simulink model "singlephaseasynchronousmotorwithFC"  (Simulink 7.3)
settings: Solver=ode45  StartTime=0.0  StopTime=0.5  RelTol=1e-3
undefined symbols (not defined in the file): Capacitor, Start
libraries: powerlib x8, simulink x2, electricdrivelib x1
settings Model: Creator=BRIG7Q  LastModifiedBy=BRIG7Q

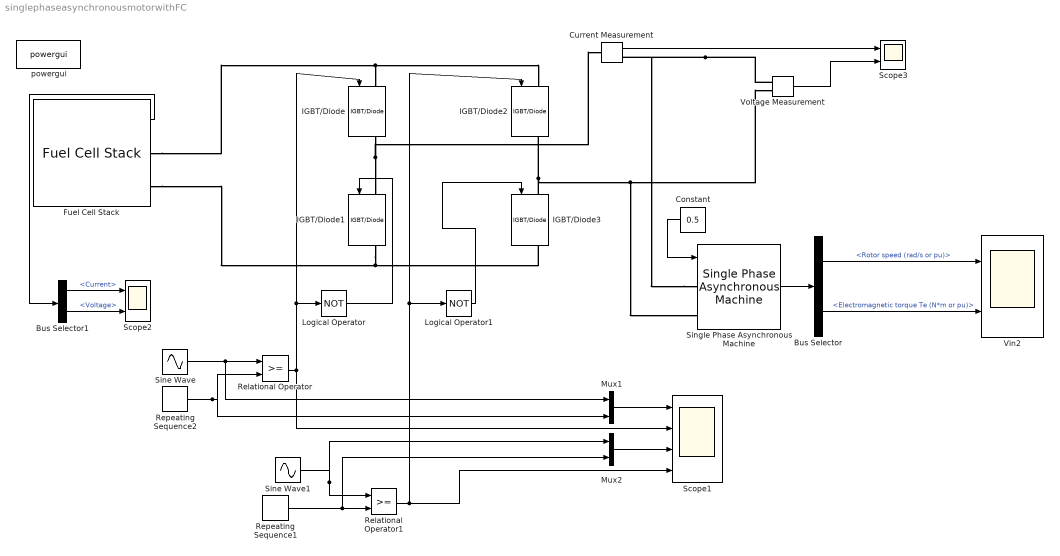
== system singlephaseasynchronousmotorwithFC ==
  Bus Selector : BusSelector  OutputSignals=Mechanical.Rotor speed (rad/s or pu),Mechanical.Electromagnetic torque Te (N*m or pu)
  Bus Selector1 : BusSelector  OutputSignals=Current,Voltage
  Constant : Constant  Value=0.5  OutDataType=fixdt(1, 16)  OutScaling=2^0
  Current Measurement : powerlib/Measurements/Current Measurement  DialogController=POWERSYS.PowerSysDialog  SystemSampleTime=-1  PhasorSimulation=off  OutputType=Complex  PSBequivalent=0
  Fuel Cell Stack : electricdrivelib/Extra Sources/Fuel Cell Stack  SystemSampleTime=-1  PresetModel=PEMFC - 1.26 kW - 24 Vdc  FcType=Proton Exchange Membrane (PEM)  Detailed=Simplified  Eoc=35  NomVI=[52, 24.23]  EndVI=[100, 20]  Nc=42  n=46  TOp=55  AirFr=2400  SuppPress=[1.5, 1]  Comp=[99.95, 21, 1]  plot_graph=off  ViewParam=off  SignX=off  SignY=off  FlowRateH2=off  FlowRateAir=off  SystemTemp=off  SystemPH2=off  SystemPAir=off  FCDyn=off  FC_tau=0
  IGBT/Diode{,1..3} (4 alike) : powerlib/Power Electronics/IGBT//Diode  DialogController=POWERSYS.PowerSysDialog  SystemSampleTime=-1  Ron=1e-3  Rs=1e5  Cs=inf  Measurements=on
  Logical Operator : Logic  Operator=NOT  AllPortsSameDT=off  OutDataTypeMode=boolean  OutDataTypeStr=boolean
  Logical Operator1 : Logic  Operator=NOT  AllPortsSameDT=off  OutDataTypeMode=boolean  OutDataTypeStr=boolean
  Mux1 : Mux  Inputs=2
  Mux2 : Mux  Inputs=2
  Relational Operator : RelationalOperator
  Relational Operator1 : RelationalOperator  LogicOutDataTypeMode=boolean  OutDataTypeStr=boolean
  Repeating Sequence1 : simulink/Sources/Repeating Sequence  SystemSampleTime=-1  rep_seq_t=[0 1/1500/4 3/1500/4 1/1500]  rep_seq_y=[0 1 -1 0]
  Repeating Sequence2 : simulink/Sources/Repeating Sequence  SystemSampleTime=-1  rep_seq_t=[0 1/1500/4 3/1500/4 1/1500]  rep_seq_y=[0 1 -1 0]
  Scope1 : Scope  NumInputPorts=4
      settings: TimeRange=0.1322916666666668  YMin=0~0~0~0  YMax=1~1~1~1
  Scope2 : Scope  NumInputPorts=2
      settings: YMin=-12.5~-45000  YMax=12.5~45000  SaveName=ScopeData3
  Scope3 : Scope  NumInputPorts=2
      settings: YMin=-12.5~-45000  YMax=12.5~45000
  Sine Wave : Sin  Amplitude=1  Bias=0  Frequency=2*pi*50  Phase=0  Samples=10  SampleTime=50e-6  Offset=0
  Sine Wave1 : Sin  Amplitude=1  Bias=0  Frequency=2*pi*50  Phase=pi  Samples=10  SampleTime=50e-6  Offset=0
  Single Phase Asynchronous Machine : powerlib/Machines/Single Phase Asynchronous Machine  DialogController=POWERSYS.PowerSysDialog  SystemSampleTime=-1  UNITS=SI  MachineType=Capacitor-Start  NominalParameters="[ .25*746  110  50]"  MainWindingStator="[2.02  7.4e-3]"  MainWindingRotor="[4.12  5.6e-3]"  MutualInductance=0.1772  AuxiliaryWinding="[7.14  8.5e-3]"  Mechanical="[0.0146  0  2 1.18]"  CapacitorStart="[2  254.7e-6]"  CapacitorRun="[18  21.1e-6]"  DisconnectionSpeed=75  InitialSpeed=0  DataType=SI  TsPowergui=0  TsBlock=-1
  Vin2 : Scope  NumInputPorts=2
      settings: YMin=0~-5  YMax=170~5  SaveName=ScopeData2
  Voltage Measurement : powerlib/Measurements/Voltage Measurement  DialogController=POWERSYS.PowerSysDialog  SystemSampleTime=-1  PhasorSimulation=off  OutputType=Complex  PSBequivalent=0
  powergui : powerlib/powergui  SystemSampleTime=-1  SimulationMode=Discrete  SampleTime=1e-6  frequency=60  SPID=off  DisableSnubberDevices=off  DisableRonSwitches=off  DisableVfSwitches=off  SwTol=0  Interpol=off  frequencyindice=0  echomessages=off  HookPort=off  DisplayEquations=off  FunctionMessages=off  EnableUseOfTLC=off  x0status=blocks  RestoreLinks=warning  Frange=[0:2:500]  Ylog=off  Xlog=on  ShowGrid=off  save=off  variable=ZData  structure=ScopeData2  ZoomFFT=off  StartTime=0.0  cycles=3  DisplayStyle=4  fundamental=50  FreqAxis=on  MaxFrequency=1000  frequencyindicesteady=1  RmsSteady=1  display=off  Ts=0  methode=off
  wires:
  Sine Wave/1 -> Relational Operator/1, Mux1/1
  Repeating Sequence2/1 -> Relational Operator/2, Mux1/2
  Relational Operator/1 -> IGBT/Diode/1, Logical Operator/1, Scope1/2
  Relational Operator1/1 -> IGBT/Diode2/1, Logical Operator1/1, Scope1/4
  Voltage Measurement/1 -> Scope3/2
  Current Measurement/1 -> Scope3/1
  Sine Wave1/1 -> Mux2/1, Relational Operator1/1
  Repeating Sequence1/1 -> Mux2/2, Relational Operator1/2
  Logical Operator/1 -> IGBT/Diode1/1
  Logical Operator1/1 -> IGBT/Diode3/1
  Mux1/1 -> Scope1/1
  Mux2/1 -> Scope1/3
  Constant/1 -> Single Phase Asynchronous Machine/1
  Single Phase Asynchronous Machine/1 -> Bus Selector/1
  Fuel Cell Stack/1 -> Bus Selector1/1
  Bus Selector1/1 -> Scope2/1  "<Current>"
  Bus Selector1/2 -> Scope2/2  "<Voltage>"
  Bus Selector/1 -> Vin2/1  "<Rotor speed (rad/s or pu)>"
  Bus Selector/2 -> Vin2/2  "<Electromagnetic torque Te (N*m or pu)>"
  connections:
  IGBT/Diode/RConn1 -- IGBT/Diode1/LConn1 -- Current Measurement/LConn1
  IGBT/Diode2/RConn1 -- Voltage Measurement/LConn2 -- Single Phase Asynchronous Machine/LConn2 -- IGBT/Diode3/LConn1
  Fuel Cell Stack/RConn1 -- IGBT/Diode2/LConn1 -- IGBT/Diode/LConn1
  Fuel Cell Stack/RConn2 -- IGBT/Diode3/RConn1 -- IGBT/Diode1/RConn1
  Single Phase Asynchronous Machine/LConn1 -- Voltage Measurement/LConn1 -- Current Measurement/RConn1
